simulink model "Universal_Bridge"  (R2021b)
settings: Solver=VariableStepAuto  StartTime=0.0  StopTime=0.2  MaxStep=1e-5  RelTol=1e-3
libraries: spsMeanLib x5, spsCurrentMeasurementLib x3, spsACVoltageSourceLib x3, spsVoltageMeasurementLib x2, spsDCMachineLib x1, spsDCVoltageSourceLib x1, spsDiodeLib x1, spsMosfetLib x1, spsPWMGeneratorDCDCLib x1, spsSeriesRLCBranchLib x1, spsUniversalBridgeLib x1, spspowerguiLib x1
settings Model: Creator=Emre Çakmakyurdu  LastModifiedBy=Emre Çakmakyurdu

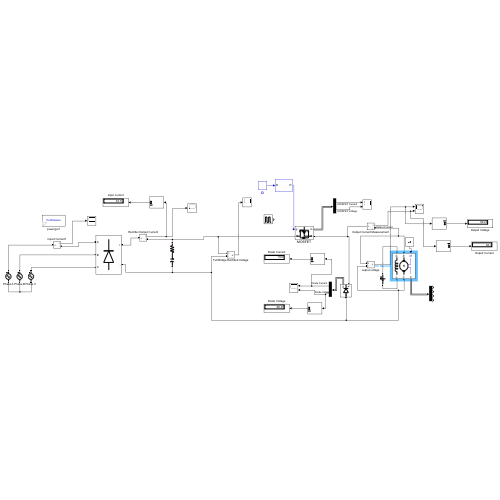
[thumbnail: Simulink's stored preview of the top-level diagram]
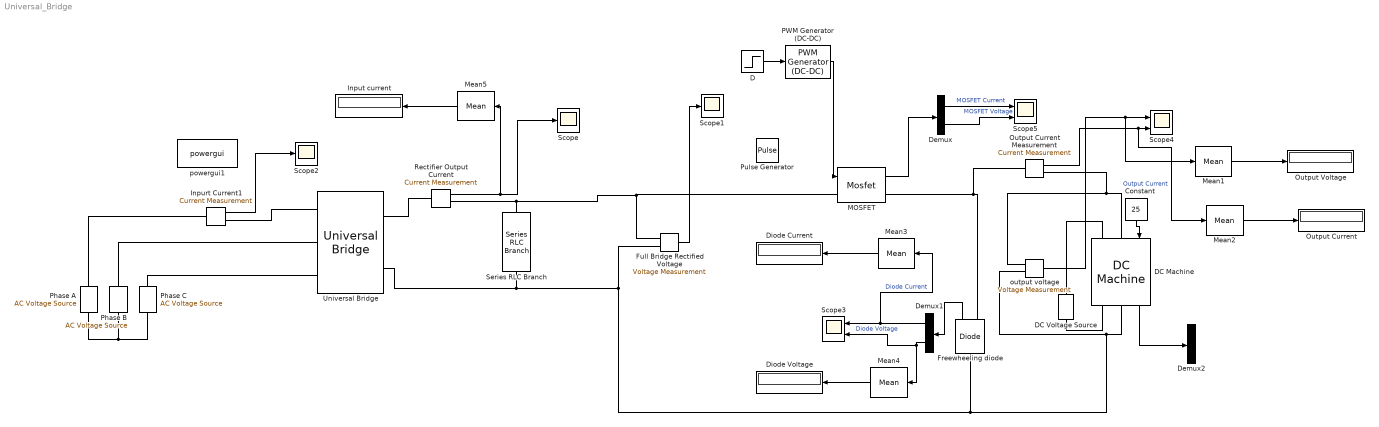
== system Universal_Bridge ==
  Constant : Constant  Value=25
  D : Step  Time=0.01  Before=0.1  After=0.4  SampleTime=0
  DC Machine : spsDCMachineLib/DC Machine  PresetModel=No  MechanicalLoad=Torque TL  FieldType=Wound  ShowDetailedParameters=on  MeasurementBus=off  RLa="[ 1.07  24.5e-3]"  RLf="[ 210  23]"  Laf=0  MachineConstant=Back-emf constant (V/rpm)  Ke=220/1500  Kt=1.8  J=1  Bm=0  Tf=0  w0=1  Ifinit=1.04761904761905  TsPowergui=0  TsBlock=-1
  DC Voltage Source : spsDCVoltageSourceLib/DC Voltage Source  Amplitude=220  Measurements=None
  Demux : Demux  Outputs=2
  Demux1 : Demux  Outputs=2
  Demux2 : Demux
  Diode Current : Display
  Diode Voltage : Display
  "Freewheeling diode " : spsDiodeLib/Diode  Ron=0  Lon=0  Vf=0  IC=0  UseSnubber=off  Rs=inf  Cs=0  Measurements=on
  Full Bridge Rectified Voltage : spsVoltageMeasurementLib/Voltage Measurement  PhasorSimulation=off  OutputType=Complex  PSBequivalent=0
  Inpurt Current1 : spsCurrentMeasurementLib/Current Measurement  PhasorSimulation=off  OutputType=Complex  PSBequivalent=0
  Input current : Display
  MOSFET : spsMosfetLib/Mosfet  Ron=0.1  Lon=0  Rd=0.01  Vfd=0  IC=0  Rs=1e5  Cs=inf  Measurements=on
  Mean{1..5} (5 alike) : spsMeanLib/Mean  Freq=50  Vinit=0  Ts=0
  Output Current : Display
  Output Current Measurement : spsCurrentMeasurementLib/Current Measurement  PhasorSimulation=off  OutputType=Complex  PSBequivalent=0
  Output Voltage : Display
  PWM Generator (DC-DC) : spsPWMGeneratorDCDCLib/PWM Generator (DC-DC)  Fsw=1e3  Ts=0
  Phase A : spsACVoltageSourceLib/AC Voltage Source  Amplitude=100*sqrt(2)  Phase=0  Frequency=50  SampleTime=0  Measurements=None  BusType=swing  Pref=10e3  Qref=0  Qmin=-inf  Qmax=+inf
  Phase B : spsACVoltageSourceLib/AC Voltage Source  Amplitude=100*sqrt(2)  Phase=-120  Frequency=50  SampleTime=0  Measurements=None  BusType=swing  Pref=10e3  Qref=0  Qmin=-inf  Qmax=+inf
  Phase C : spsACVoltageSourceLib/AC Voltage Source  Amplitude=100*sqrt(2)  Phase=120  Frequency=50  SampleTime=0  Measurements=None  BusType=swing  Pref=10e3  Qref=0  Qmin=-inf  Qmax=+inf
  Pulse Generator : DiscretePulseGenerator  PulseType=Time based  Period=1/1000  PulseWidth=80
  Rectifier Output Current : spsCurrentMeasurementLib/Current Measurement  PhasorSimulation=off  OutputType=Complex  PSBequivalent=0
  Scope : Scope
  Scope1 : Scope
  Scope2 : Scope
  Scope3 : Scope  NumInputPorts=2
  Scope4 : Scope  NumInputPorts=2
  Scope5 : Scope  NumInputPorts=2
  Series RLC Branch : spsSeriesRLCBranchLib/Series RLC Branch  LConnTagsString=__new0  RConnTagsString=__new0  BranchType=RC  Resistance=1e-4  Inductance=1e-3  SetiL0=off  InitialCurrent=0  Capacitance=1e-4  Setx0=off  InitialVoltage=0  Measurements=None
  Universal Bridge : spsUniversalBridgeLib/Universal Bridge  Arms=3  SnubberResistance=inf  SnubberCapacitance=0  Device=Diodes  Ron=0  Lon=0  ForwardVoltages="[  0  0  ]"  ForwardVoltage=0  GTOparameters=[ 10e-6 , 20e-6 ]  IGBTparameters=[ 1e-6 , 2e-6 ]  Measurements=None  Measurements_2=None  converterType=Rectifier
  output voltage : spsVoltageMeasurementLib/Voltage Measurement  PhasorSimulation=off  OutputType=Complex  PSBequivalent=0
  powergui1 : spspowerguiLib/powergui  Priority=1  SimulationMode=Continuous  SampleTime=50e-6  frequency=60  Iterations=50  frequencyindice=50  Pbase=100e6  ErrMax=1e-4  UnitsV=kV  UnitsW=MW  buscounter=0  FunctionMessages=off  echomessages=off  EnableUseOfTLC=off  CurrentSourceSwitches=off  DisableSnubberDevices=off  DisableRonSwitches=off  DisableVfSwitches=off  DisplayEquations=off  AutomaticDiscreteSolvers=off  SolverType=Tustin/Backward Euler (TBE)  Interpol=off  ExternalGateDelay=off  methode=off  Ts=100  x0status=blocks  SPID=on  SwTol=0  HookPort=off  NonlinearTolerance=1e-4  nMaxIteration=100  ContinueOnMaxIteration=off  RestoreLinks=warning  ResistiveCurrentMeasurement=off  Frange=[0:2:500]  Ylog=off  Xlog=on  ShowGrid=off  save=off  variable=ZData  structure=0  ZoomFFT=off  StartTime=0.0  cycles=1  DisplayStyle=1  fundamental=60  FreqAxis=off  MaxFrequency=1000  frequencyindicesteady=1  RmsSteady=1  display=off
  wires:
  Rectifier Output Current/1 -> Mean5/1, Scope/1
  Full Bridge Rectified Voltage/1 -> Scope1/1
  Inpurt Current1/1 -> Scope2/1
  Demux1/1 -> Mean3/1, Scope3/1  "Diode Current"
  "Freewheeling diode "/1 -> Demux1/1
  MOSFET/1 -> Demux/1
  Mean3/1 -> Diode Current/1
  Demux1/2 -> Mean4/1, Scope3/2  "Diode Voltage"
  Mean4/1 -> Diode Voltage/1
  Constant/1 -> DC Machine/1
  DC Machine/1 -> Demux2/1
  Output Current Measurement/1 -> Mean2/1, Scope4/2  "Output Current"
  output voltage/1 -> Mean1/1, Scope4/1
  Demux/1 -> Scope5/1  "MOSFET Current"
  Demux/2 -> Scope5/2  "MOSFET Voltage"
  Mean1/1 -> Output Voltage/1
  Mean2/1 -> Output Current/1
  Mean5/1 -> Input current/1
  D/1 -> PWM Generator (DC-DC)/1
  PWM Generator (DC-DC)/1 -> MOSFET/1
  connections:
  Phase B/RConn1 -- Universal Bridge/LConn2
  Phase C/RConn1 -- Universal Bridge/LConn3
  Phase C/LConn1 -- Phase B/LConn1 -- Phase A/LConn1
  Full Bridge Rectified Voltage/LConn1 -- MOSFET/LConn1 -- Rectifier Output Current/RConn1 -- Series RLC Branch/LConn1
  Universal Bridge/RConn2 -- output voltage/LConn2 -- DC Machine/RConn1 -- "Freewheeling diode "/LConn1 -- Full Bridge Rectified Voltage/LConn2 -- Series RLC Branch/RConn1
  Rectifier Output Current/LConn1 -- Universal Bridge/RConn1
  Phase A/RConn1 -- Inpurt Current1/LConn1
  Inpurt Current1/RConn1 -- Universal Bridge/LConn1
  MOSFET/RConn1 -- "Freewheeling diode "/RConn1 -- Output Current Measurement/LConn1
  DC Machine/LConn1 -- output voltage/LConn1 -- Output Current Measurement/RConn1
  DC Voltage Source/RConn1 -- DC Machine/LConn2
  DC Machine/RConn2 -- DC Voltage Source/LConn1
